simulink model "new_dynamics_sim"  (R2024b)
settings: Solver=VariableStepAuto  StartTime=0.0  StopTime=1  RelTol=1e-3
values from neighbouring files (symbols this model uses):
  A = [0 1 ... (first row only)    [dynamics_transfer_function.m]
  B = [0; b]    [dynamics_transfer_function.m]
  C = [1 0]    [dynamics_transfer_function.m]
  D = 0    [dynamics_transfer_function.m]
  G = (( s + 40 ) / ( s + 400 ))    [new_dynamics.m]
  k = 7e3    (= 7000)    [new_dynamics.m]
  P1 = ( 1/L ) / ( s + R/L )    [new_dynamics.m]
  P2 = ( b ) / ( s^2 - a )    [new_dynamics.m]
  sys_d = c2d(G, Ts)    [new_dynamics.m]
settings Model: Creator=shara  LastModifiedBy=shara

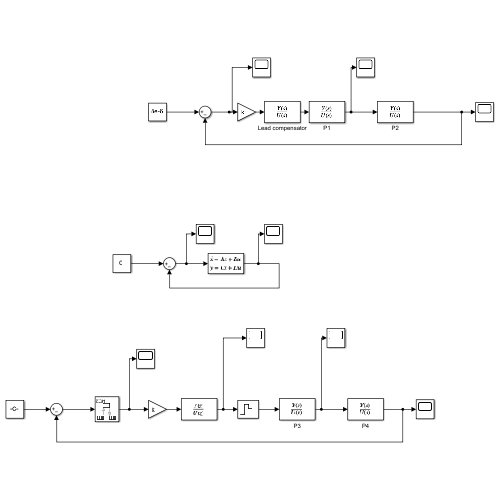
[thumbnail: Simulink's stored preview of the top-level diagram]
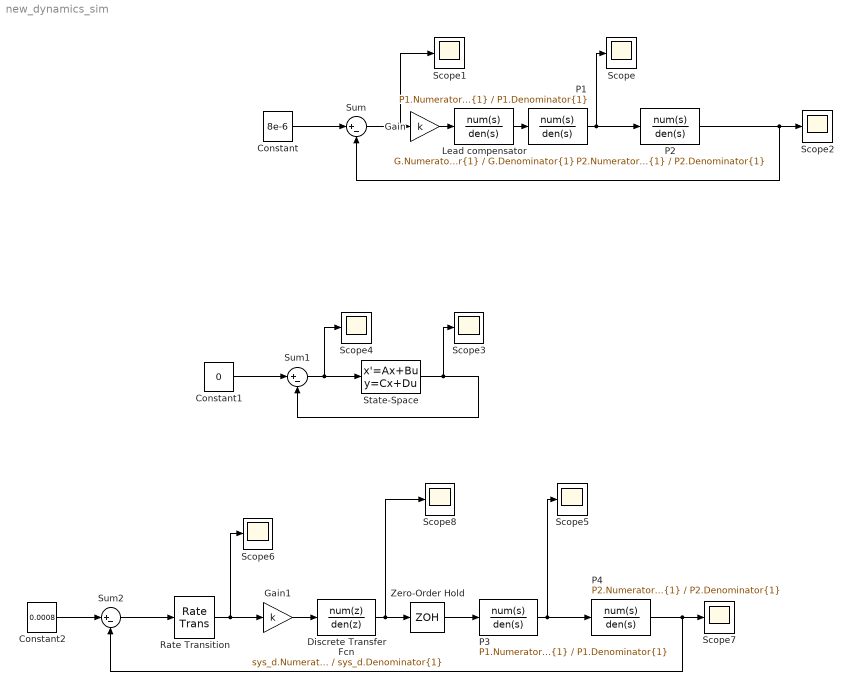
== system new_dynamics_sim ==
  Constant : Constant  Value=8e-6
  Constant1 : Constant  Value=0
  Constant2 : Constant  Value=0.0008
  Discrete Transfer Fcn : DiscreteTransferFcn  Numerator=sys_d.Numerator{1}  Denominator=sys_d.Denominator{1}
  Gain : Gain  Gain=k
  Gain1 : Gain  Gain=k
  Lead compensator : TransferFcn  Numerator=G.Numerator{1}  Denominator=G.Denominator{1}
  P1 : TransferFcn  Numerator=P1.Numerator{1}  Denominator=P1.Denominator{1}
  P2 : TransferFcn  Numerator=P2.Numerator{1}  Denominator=P2.Denominator{1}
  P3 : TransferFcn  Numerator=P1.Numerator{1}  Denominator=P1.Denominator{1}
  P4 : TransferFcn  Numerator=P2.Numerator{1}  Denominator=P2.Denominator{1}
  Rate Transition : RateTransition  OutPortSampleTime=1e-3
  Scope{,1..8} (9 alike) : Scope
  State-Space : StateSpace  A=A  B=B  C=C  D=D  InitialCondition=[0.01 0 0 0]
  Sum : Sum  Inputs=|+-
  Sum1 : Sum  Inputs=|+-
  Sum2 : Sum  Inputs=|+-
  Zero-Order Hold : ZeroOrderHold  SampleTime=1e-3
  wires:
  P1/1 -> P2/1, Scope/1
  Constant/1 -> Sum/1
  Sum/1 -> Scope1/1, Gain/1
  Gain/1 -> Lead compensator/1
  Lead compensator/1 -> P1/1
  P2/1 -> Sum/2, Scope2/1
  Constant1/1 -> Sum1/1
  Sum1/1 -> Scope4/1, State-Space/1
  State-Space/1 -> Scope3/1, Sum1/2
  P3/1 -> P4/1, Scope5/1
  Constant2/1 -> Sum2/1
  Discrete Transfer Fcn/1 -> Scope8/1, Zero-Order Hold/1
  Gain1/1 -> Discrete Transfer Fcn/1
  P4/1 -> Scope7/1, Sum2/2
  Rate Transition/1 -> Scope6/1, Gain1/1
  Zero-Order Hold/1 -> P3/1
  Sum2/1 -> Rate Transition/1
